simulink model "test_pedal_wheel_animation"  (Simulink 4.00)
settings: Solver=ode1  StartTime=0.0  StopTime=60  FixedStep=0.05  RelTol=1e-3
libraries: pedal_wheel_animation_lib x1, simulink3 x1
settings Model: LastModifiedBy=bsaunder  RTWOptions="-aEnforceIntegerDowncast=1 -aExtMode=0 -aFoldNonRolledExpr=1 -aForceParamTrailComments=0 -aGenerateComments=1 -aIgnoreCustomStorageClasses=0 -aIncHierarchyInIds=0 -aInlineInvariantSignals=0 -aLocalBlockOutputs=1 -aLogVarNameModifier=\"rt_\" -aRTWVerbose=1 -aRollThreshold=5 -aShowEliminatedStatements=1"

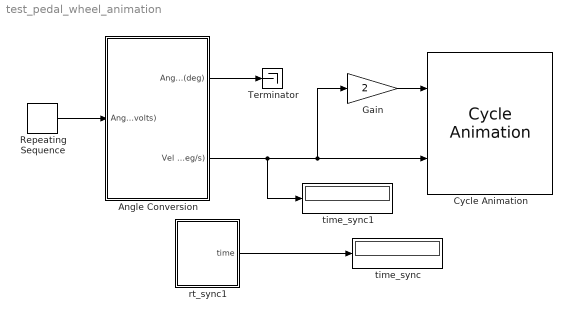
== system test_pedal_wheel_animation ==
  Angle Conversion : Subsystem
      settings: RTWFcnNameOpts=Auto  RTWFileNameOpts=Auto
  Cycle Animation : pedal_wheel_animation_lib/Cycle Animation  show=on  Ts=0.05
  Gain : Gain  Gain=2  Multiplication=Element-wise(K.*u)  SaturateOnIntegerOverflow=on
  Repeating Sequence : simulink3/Sources/Repeating Sequence  rep_seq_t=[0 20 40 60]  rep_seq_y=[0.0 0.2 0.5 1.0]
  Terminator : Terminator
  rt_sync1 : Subsystem  mask{Ts=0.05}
      mask prompts: Ts "Sample Time"
      settings: RTWFcnNameOpts=Auto  RTWFileNameOpts=Auto
      mask Display: fprintf('Real\n Time\n sync')
  time_sync : Display
      settings: Format=short
  time_sync1 : Display
      settings: Format=short
  wires:
  rt_sync1/1(time) -> time_sync/1
  Repeating Sequence/1 -> Angle Conversion/1(Angle (0 to 1 volts))
  Angle Conversion/2(Vel (deg/s)) -> Gain/1, Cycle Animation/2, time_sync1/1
  Gain/1 -> Cycle Animation/1
  Angle Conversion/1(Angle (deg)) -> Terminator/1

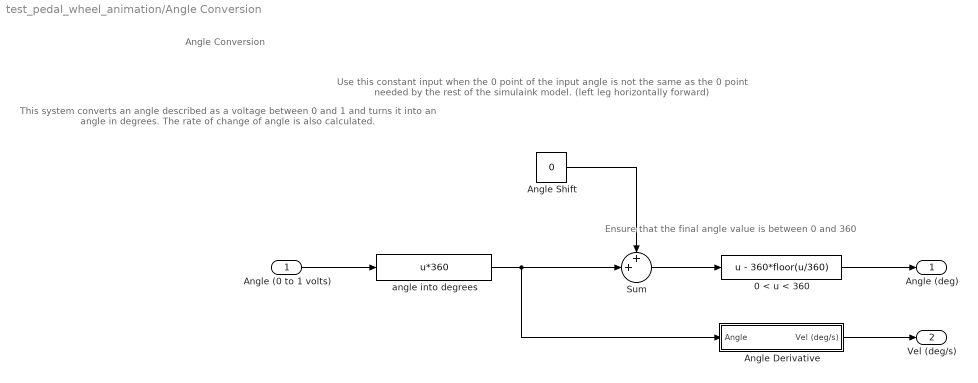
== system test_pedal_wheel_animation/Angle Conversion ==
  note: Ensure that the final angle
      | value is between 0 and 360
  note: This system converts an
      | angle described as a voltage
      | between 0 and 1 and turns it
      | into an angle in degrees.
      | The rate of change of angle
      | is also calculated.
  note: Use this constant input
      | when the 0 point of the
      | input angle is not the same
      | as the 0 point needed by
      | the rest of the simulaink
      | model.
      | (left leg horizontally forward)
  note: Angle Conversion
  Angle (0 to 1 volts) : Inport  Port=1  LatchInput=off
  0 < u < 360 : Fcn  Expr=u - 360*floor(u/360)
  Angle Derivative : Subsystem  mask(AngleDer){Tdf=0.5, Ts=0.05}
      mask prompts: Tdf "Filter constant"; Ts "Sampling Time"
      mask help:
      | This block calculates the angular velocity from the angle measuremet.  If the input angle is in degrees then the output velocity is in deg/s.  The block takes account of the transition from 359 deg to 0 deg or vice versa and computes the derivative based on the sample time given  The output is passed through a low pass filter based on the fliter constant also given.
      |
      | Implemented by Nils-Otto Negaard
      | Documented by Ben Saunders (17/06/2003)
      settings: RTWFcnNameOpts=Auto  RTWFileNameOpts=Auto
  Angle Shift : Constant  Value=0
  Sum : Sum  Inputs=++|  SaturateOnIntegerOverflow=on
  angle into degrees : Fcn  Expr=u*360
  Angle (deg) : Outport  Port=1
  Vel (deg/s) : Outport  Port=2
  wires:
  Angle Derivative/1(Vel (deg/s)) -> Vel (deg/s)/1
  Angle (0 to 1 volts)/1 -> angle into degrees/1
  0 < u < 360/1 -> Angle (deg)/1
  Sum/1 -> 0 < u < 360/1
  angle into degrees/1 -> Sum/2, Angle Derivative/1(Angle)
  Angle Shift/1 -> Sum/1

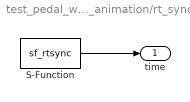
== system test_pedal_wheel_animation/rt_sync1 ==
  S-Function : S-Function  FunctionName=sf_rtsync  Parameters=Ts  PortCounts=[]  SFunctionModules=''
  time : Outport  Port=1
  wires:
  S-Function/1 -> time/1

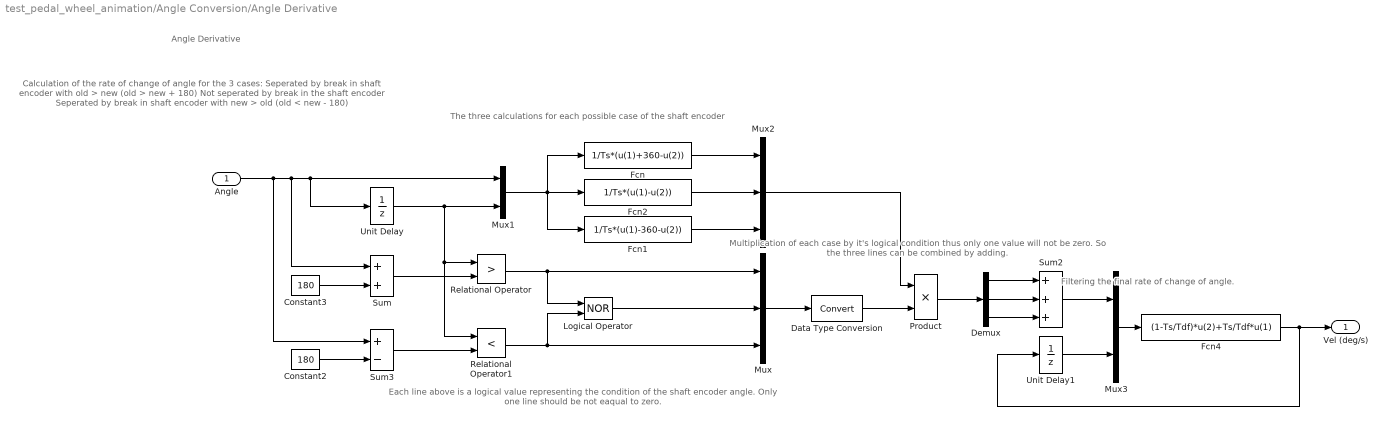
== system test_pedal_wheel_animation/Angle Conversion/Angle Derivative ==
  note: Angle Derivative
  note: Filtering the final rate of
      | change of angle.
  note: Multiplication of each case
      | by it's logical condition thus
      | only one value will not be zero.
      | So the three lines can be
      | combined by adding.
  note: The three calculations for each
      | possible case of the shaft encoder
  note: Each line above is a logical value
      | representing the condition of the
      | shaft encoder angle.  Only one line
      | should be not eaqual to zero.
  note: Calculation of the rate of change of angle
      | for the 3 cases:
      | Seperated by break in shaft encoder with old > new (old > new + 180)
      | Not seperated by break in the shaft encoder
      | Seperated by break in shaft encoder with new > old (old < new - 180)
  Angle : Inport  Port=1  LatchInput=off
  Constant2 : Constant  Value=180  VectorParams1D=off
  Constant3 : Constant  Value=180  VectorParams1D=off
  Data Type Conversion : DataTypeConversion  DataType=double  SaturateOnIntegerOverflow=on
  Demux : Demux  Outputs=3  BusSelectionMode=off
  Fcn : Fcn  Expr=1/Ts*(u(1)+360-u(2))
  Fcn1 : Fcn  Expr=1/Ts*(u(1)-360-u(2))
  Fcn2 : Fcn  Expr=1/Ts*(u(1)-u(2))
  Fcn4 : Fcn  Expr=(1-Ts/Tdf)*u(2)+Ts/Tdf*u(1)
  Logical Operator : Logic  Operator=NOR  Inputs=2
  Mux : Mux  Inputs=3
  Mux1 : Mux  Inputs=2
  Mux2 : Mux  Inputs=3
  Mux3 : Mux  Inputs=2
  Product : Product  Inputs=2  Multiplication=Element-wise(.*)  SaturateOnIntegerOverflow=on
  Relational Operator : RelationalOperator  Operator=>
  Relational Operator1 : RelationalOperator  Operator=<
  Sum : Sum  Inputs=++  SaturateOnIntegerOverflow=on
  Sum2 : Sum  Inputs=+++  SaturateOnIntegerOverflow=on
  Sum3 : Sum  Inputs=+-  SaturateOnIntegerOverflow=on
  Unit Delay : UnitDelay  X0=0  SampleTime=0.05
      settings: RTWStateStorageClass=Auto
  Unit Delay1 : UnitDelay  X0=0  SampleTime=Ts
      settings: RTWStateStorageClass=Auto
  Vel (deg/s) : Outport  Port=1
  wires:
  Fcn1/1 -> Mux2/3
  Fcn2/1 -> Mux2/2
  Logical Operator/1 -> Mux/2
  Sum3/1 -> Relational Operator1/2
  Constant3/1 -> Sum/2
  Angle/1 -> Unit Delay/1, Mux1/1, Sum/1, Sum3/1
  Sum2/1 -> Mux3/1
  Demux/3 -> Sum2/3
  Demux/2 -> Sum2/2
  Demux/1 -> Sum2/1
  Product/1 -> Demux/1
  Unit Delay1/1 -> Mux3/2
  Mux3/1 -> Fcn4/1
  Fcn4/1 -> Vel (deg/s)/1, Unit Delay1/1
  Mux2/1 -> Product/1
  Fcn/1 -> Mux2/1
  Mux1/1 -> Fcn2/1, Fcn1/1, Fcn/1
  Mux/1 -> Data Type Conversion/1
  Relational Operator/1 -> Mux/1, Logical Operator/1
  Relational Operator1/1 -> Mux/3, Logical Operator/2
  Constant2/1 -> Sum3/2
  Sum/1 -> Relational Operator/2
  Unit Delay/1 -> Relational Operator/1, Relational Operator1/1, Mux1/2
  Data Type Conversion/1 -> Product/2
